simulink model "ClarkePark"  (Simulink 6.4)
settings: Solver=ode45  StartTime=0.0  StopTime=100e-3  RelTol=1e-3
settings Model: LastModifiedBy=Daniel

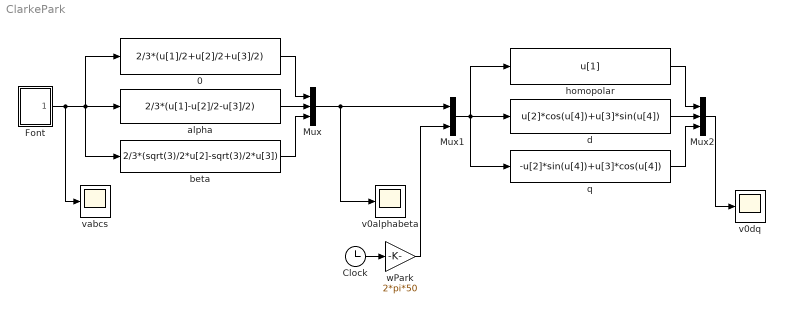
== system ClarkePark ==
  0 : Fcn  Expr=2/3*(u[1]/2+u[2]/2+u[3]/2)
  Clock : Clock
      settings: Decimation=10
  Font : Subsystem
  Mux : Mux  Inputs=3
  Mux1 : Mux  Inputs=2
  Mux2 : Mux  Inputs=3
  alpha : Fcn  Expr=2/3*(u[1]-u[2]/2-u[3]/2)
  beta : Fcn  Expr=2/3*(sqrt(3)/2*u[2]-sqrt(3)/2*u[3])
  d : Fcn  Expr=u[2]*cos(u[4])+u[3]*sin(u[4])
  homopolar : Fcn  Expr=u[1]
  q : Fcn  Expr=-u[2]*sin(u[4])+u[3]*cos(u[4])
  v0alphabeta : Scope
  v0dq : Scope
      settings: SaveName=ScopeData2
  vabcs : Scope
  wPark : Gain  Gain=2*pi*50
  wires:
  Font/1(vabcs) -> vabcs/1, alpha/1, beta/1, 0/1
  0/1 -> Mux/1
  alpha/1 -> Mux/2
  beta/1 -> Mux/3
  Mux/1 -> v0alphabeta/1, Mux1/1
  Clock/1 -> wPark/1
  wPark/1 -> Mux1/2
  Mux1/1 -> d/1, q/1, homopolar/1
  homopolar/1 -> Mux2/1
  d/1 -> Mux2/2
  q/1 -> Mux2/3
  Mux2/1 -> v0dq/1

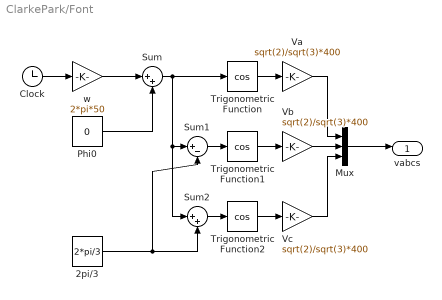
== system ClarkePark/Font ==
  2pi/3 : Constant  Value=2*pi/3  OutDataType=sfix(16)  ConRadixGroup=Use specified scaling  OutScaling=2^0  SampleTime=inf  FramePeriod=inf
  Clock : Clock
      settings: Decimation=10
  Mux : Mux  Inputs=3
  Phi0 : Constant  Value=0  OutDataType=sfix(16)  ConRadixGroup=Use specified scaling  OutScaling=2^0  SampleTime=inf  FramePeriod=inf
  Sum : Sum  Inputs=|++
  Sum1 : Sum  Inputs=|+-
  Sum2 : Sum  Inputs=|++
  Trigonometric Function : Trigonometry  Operator=cos
  Trigonometric Function1 : Trigonometry  Operator=cos
  Trigonometric Function2 : Trigonometry  Operator=cos
  Va : Gain  Gain=sqrt(2)/sqrt(3)*400
  Vb : Gain  Gain=sqrt(2)/sqrt(3)*400
  Vc : Gain  Gain=sqrt(2)/sqrt(3)*400
  w : Gain  Gain=2*pi*50
  vabcs : Outport
  wires:
  Clock/1 -> w/1
  w/1 -> Sum/1
  Phi0/1 -> Sum/2
  Sum/1 -> Trigonometric Function/1, Sum1/1, Sum2/1
  2pi/3/1 -> Sum2/2, Sum1/2
  Sum1/1 -> Trigonometric Function1/1
  Sum2/1 -> Trigonometric Function2/1
  Trigonometric Function/1 -> Va/1
  Trigonometric Function1/1 -> Vb/1
  Trigonometric Function2/1 -> Vc/1
  Mux/1 -> vabcs/1
  Va/1 -> Mux/1
  Vb/1 -> Mux/2
  Vc/1 -> Mux/3
